simulink model "dfig_dtc_ann"  (R2014a)
settings: Solver=ode23tb  StartTime=0.0  StopTime=10.0  RelTol=1e-3
libraries: neural x106, powerlib x11, powerlib_meascontrol x5, simulink x1
(part 3 of 3)

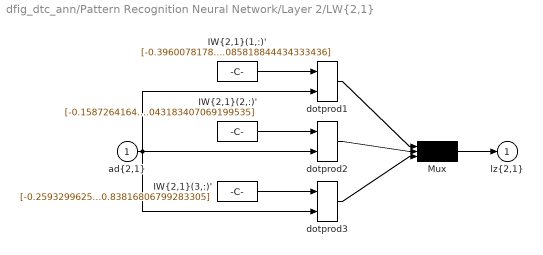
== system dfig_dtc_ann/Pattern Recognition Neural Network/Layer 2/LW{2,1} ==
  "ad{2,1}" : Inport  PortDimensions=100
      mask Display: e = 0.06;c1 = [120 230 180]/255;c2 = ([120 230 180]+0)/(256+128);c3 = ([120 230 180]+128)/(256+128);patch([0 1 1 0],[0 0 1 1],c1);patch([0 1 1 1-e 1-e 0+e],[0 0 1 1-e 0+e 0+e],c2);patch([0 0 1 1-e 0+e 0+e],[0 1 1 1-e 1-e 0+e],c3);plot([0 1 1 0 0],[0 0 1 1 0]);
  "IW{2,1}(1,:)'" : Constant  Value=[-0.39600781788832012;0.80103533096718704;0.41301121989245843;1.1771326908066198;-0.72135382694368677;-0.28776648831982082;0.1961289184675187;1.1440764500026632;-0.23525252157370444;-0.6157189814984334;-0.40248389897597353;-0.4661359120182772;-1.1436532688880334;0.36554497438624434;0.35212901502733357;-1.0882332208589625;0.32805995130326643;-0.37938264281970058;-0.14182705379747199;0.24958969950995402;-0.10265993569030581;0.28425296840325154;-0.32357116420013993;-0.094829576525869916;0.79951067009868138;0.34584911554053616;1.0427282838344432;0.83831785938073644;0.44529056694505259;-0.32121203525474484;0.47873089139593306;0.39423469234562103;-0.13128858500573656;0.92671664955040856;0.045646817038878865;-0.12672354804290886;-0.086421412067187328;0.57657556928792952;-0.062468935112063043;0.26127992146476609;0.34916854352459359;0.39828802839161381;0.76429667962811487;0.22808333560465002;-0.81115136059134063;0.53620443728919553;0.38872445822292429;-0.014891697234410965;0.089173483711878096;0.47345534641936177;-0.71425698724277542;-0.41530443422428559;-0.16469285817743728;-0.37393482186322324;0.18530095941638727;0.64898422181938475;0.09192495445191208;-1.2135091283197963;0.022857999255296524;-0.061188709760653402;0.3432789805346092;0.48379081701553334;-0.11894930315772172;0.017970627109767028;-0.36966997740729218;-0.17616356039153838;0.68742042155939309;0.21297253162193769;0.26859586653067541;-0.37911756178809991;-0.31892610288538376;0.54184108935259523;0.0075175193083964007;-0.29962602080773765;0.56464120152362596;-0.086909709470131366;0.69356886662087025;0.83865301224458633;-0.50614592854819307;-0.1669266161112779;0.61967502129516694;-0.70389310289164331;-0.97647889962465872;0.58839307925056816;-1.2405837996232545;0.30913121120624376;0.44417213686044177;0.85448116388694384;-0.72952901034177886;0.53358762615259592;0.7277496647025159;-0.47770579297136512;0.065512285355189409;-0.024696170024412128;0.33184400224384625;0.77506264674556313;0.14747927143471062;-0.064782569224002454;1.1987950072029985;0.085818844434333436]
      mask Display: e = 0.06;c1 = [120 150 230]/255;c2 = ([120 150 230]+0)/383;c3 = ([120 150 230]+128)/383;patch([0 1 1 0],[0 0 1 1],c1);patch([0 1 1 1-e 1-e 0+e],[0 0 1 1-e 0+e 0+e],c2);patch([0 0 1 1-e 0+e 0+e],[0 1 1 1-e 1-e 0+e],c3);plot([0 1 1 0 0],[0 0 1 1 0]);disp('weights');
  "IW{2,1}(2,:)'" : Constant  Value=[-0.15872641642325955;0.25485844916090572;-0.13632880124207802;-1.0522862221388374;0.012548262724917304;0.050580761236192887;-0.80496802803384571;0.19867650282491883;-0.91745965435057808;-0.84257241706486619;0.065899167127548175;0.54758998719824958;-0.12769643438691047;-0.20898168594609567;-0.64094433173500898;-0.65626789120602724;0.9378120797035765;0.93741066325888078;-0.1115824055347789;0.36549095652773905;0.11096813586489501;0.42307687617734807;-0.36669342329534288;0.82844283524153506;-0.8696511847899131;-0.44266645748114508;-0.21416027683746078;0.11931881155251664;0.82053660406186268;-0.030940761976304361;-0.43271567557985519;1.3438050326709607;0.24153096743304692;0.47835126648124704;-0.72516632400891712;1.0406552999708416;0.53219988971029786;1.6428530389630933;-0.34613733337427577;1.3382882669797933;-0.050102330938810717;0.36085160506818409;0.33183575113754571;-0.21614196040392783;-0.55735322710081481;-0.58225353209158204;0.36550444844041868;0.92056698514446278;-0.26814264333390131;0.64990851258155902;0.6422471733856121;-0.42842320458710942;-0.3550641155339887;0.22066080403826688;-0.48815244166069616;0.72941025675976423;0.51283736806009617;-0.3534937499750086;-1.3312389260991802;-0.39518675849242418;0.78872014932885415;0.35575719119600263;-0.042002321801973025;-1.114402874237632;-0.63378154148624721;-0.23841783841595648;0.56659938013089528;0.20205621739426555;0.19221934898095491;0.11557327779329152;0.75738433485393852;0.82456230330850788;-0.21497552250640226;0.43042182568864623;0.67330144504280764;-0.10709263657939555;0.35267493092517049;0.62842610467547266;-0.33229774822208258;-0.69561342086413736;-0.98378004697372901;-0.17510423116292634;-0.010675115122412697;-0.36995663381985;-0.23043337938054204;-0.13343865366168817;0.39523416686265067;-0.83041390827011785;0.13579111643546179;0.79961703337559364;-0.11902985188294168;-0.099737720935565211;-0.82220442849952646;-0.59133131984649467;-0.013397692495460717;-0.30409995119193683;-0.050800794187225912;-0.58357949953185295;-0.53366952839260839;0.043183407069199535]
      mask Display: e = 0.06;c1 = [120 150 230]/255;c2 = ([120 150 230]+0)/383;c3 = ([120 150 230]+128)/383;patch([0 1 1 0],[0 0 1 1],c1);patch([0 1 1 1-e 1-e 0+e],[0 0 1 1-e 0+e 0+e],c2);patch([0 0 1 1-e 0+e 0+e],[0 1 1 1-e 1-e 0+e],c3);plot([0 1 1 0 0],[0 0 1 1 0]);disp('weights');
  "IW{2,1}(3,:)'" : Constant  Value=[-0.25932996251483764;-0.45562444180686124;0.082585767141114902;0.83272636912942721;0.59433907990150692;0.55001151242535062;-0.56259714883901957;-0.62797492129839039;-0.25938685852771254;-0.058217758000340167;0.044223075395425242;-0.23477610476758989;0.52283195141505323;0.89505974868488569;-0.20701295215162463;0.66816935702873281;0.098098587269625781;0.029573975414518085;0.88218211179692074;0.36073579489144675;-0.40744885981040091;0.092101970169830544;-0.46564910869122011;0.12812380140714019;-1.2827155630720604;0.69695621757152382;0.30812061678832425;0.79767265701525303;0.17672573541318648;-0.54955370831702322;0.033619925789093848;0.49346621662848372;0.56630037710386594;-0.78758323442448408;-0.055222376284757846;0.90928269805545514;-0.12908860635657129;0.42838783825163473;-0.41076812833442228;0.56237657135593522;-0.68700671917372402;-0.64758082415616292;0.99331324379955122;0.23297084258953685;-0.020654675763786677;0.83855505303753397;-0.3252122104798541;0.37193247898627541;-0.10662297511608393;0.51474873965120072;-0.66419405396046727;0.58280501519241523;-0.6526494783117136;0.1216061925420038;-0.078507863021873334;0.28319403079758726;-0.87218346967029692;-0.81577283653680288;-0.41636369589804462;-0.98003924590756508;0.7973673695014436;0.40291242287379286;-0.2867637365923269;0.99759735322669163;0.65834762569595617;1.0678820008485042;-0.23775717257239001;0.084590844274157445;0.41132861031693563;-0.36074025256143272;0.58957921516273259;-0.84150388421390976;-0.33218145349908124;0.23583393588002838;-0.3825655887183963;0.42631617144173894;-0.32964074775802482;0.40295677014248082;0.018782930942609556;-0.66064472557358389;0.79119426329714626;0.37364326884475485;-0.18924863509760317;-0.56498056843220334;-1.0720533763733813;0.59388182732315176;-0.87601519091150082;0.04206405522411967;-0.9920496692258769;0.73122033113882579;-0.08167381081958161;-0.034139549187767876;0.77158401935233578;0.86919728299791199;0.62762726668100355;0.42415120492076525;0.43647371945047997;0.019170076695867701;-0.89256756698482964;-0.83816806799283305]
      mask Display: e = 0.06;c1 = [120 150 230]/255;c2 = ([120 150 230]+0)/383;c3 = ([120 150 230]+128)/383;patch([0 1 1 0],[0 0 1 1],c1);patch([0 1 1 1-e 1-e 0+e],[0 0 1 1-e 0+e 0+e],c2);patch([0 0 1 1-e 0+e 0+e],[0 1 1 1-e 1-e 0+e],c3);plot([0 1 1 0 0],[0 0 1 1 0]);disp('weights');
  Mux : Mux  Inputs=3
      mask Display: e = 0.06;c1 = [120 150 230]/255;c2 = ([120 150 230]+0)/383;c3 = ([120 150 230]+128)/383;patch([0 1 1 0],[0 0 1 1],c1);patch([0 1 1 1-e 1-e 0+e],[0 0 1 1-e 0+e 0+e],c2);patch([0 0 1 1-e 0+e 0+e],[0 1 1 1-e 1-e 0+e],c3);plot([0 1 1 0 0],[0 0 1 1 0]);disp('Mux');
  dotprod1 : neural/Weight Functions/dotprod
  dotprod2 : neural/Weight Functions/dotprod
  dotprod3 : neural/Weight Functions/dotprod
  "lz{2,1}" : Outport
      mask Display: e = 0.06;c1 = [120 230 180]/255;c2 = ([120 230 180]+0)/(256+128);c3 = ([120 230 180]+128)/(256+128);patch([0 1 1 0],[0 0 1 1],c1);patch([0 1 1 1-e 1-e 0+e],[0 0 1 1-e 0+e 0+e],c2);patch([0 0 1 1-e 0+e 0+e],[0 1 1 1-e 1-e 0+e],c3);plot([0 1 1 0 0],[0 0 1 1 0]);
  wires:
  "IW{2,1}(1,:)'"/1 -> dotprod1/1
  "ad{2,1}"/1 -> dotprod1/2, dotprod2/2, dotprod3/2
  dotprod1/1 -> Mux/1
  "IW{2,1}(2,:)'"/1 -> dotprod2/1
  dotprod2/1 -> Mux/2
  "IW{2,1}(3,:)'"/1 -> dotprod3/1
  dotprod3/1 -> Mux/3
  Mux/1 -> "lz{2,1}"/1

== matlab function dfig_dtc_ann/Two-Level Hystereis Band ==
  data: FluxRef input; Hf output; Flux input; m input; mm output
function [Hf,mm] = Two_Level_Hys(FluxRef,Flux,m)
 
DelF=0.025;% Hysteresis Width for Flux
Hf=0;%Initializing Hysteresis Controller Output For Flux
mm=m;
% Flux Two Level Hysteresis Band %
%------------------------------------------------------------------------%
if(Flux<=(FluxRef-DelF))
    Hf=1;
    mm=Hf;
end
if(mm==1&&(Flux>(FluxRef-DelF))&&(Flux<(FluxRef+DelF)))
    Hf=1;
    mm=Hf;
end
if(Flux>=(FluxRef+DelF))
    Hf=0;
    mm=Hf;
end
if(mm==0&&(Flux>(FluxRef-DelF))&&(Flux<(FluxRef+DelF)))
    Hf=0;
    mm=Hf;
end

== matlab function dfig_dtc_ann/Rotor Flux Torque Estimator (4) ==
  data: Sird input; SirMag output; Sirq input; Irq input; Sisd input; SirAng output; Torque output
function [SirMag,SirAng,Torque] = Rotor_Flux_Torque_Estimator(Sird,Sirq,Irq,Sisd)
 SirMag=((Sird)^(2)+(Sirq)^(2))^(0.5);
 x=atan2(Sirq,Sird);
 if(x>=0)
    SirAng=x*(180/pi);
 else
    SirAng=x*(180/pi)+360;
 end
 Torque=(-3)*(0.0135/0.0136)*(Sisd*Irq);

== matlab function dfig_dtc_ann/Stator Flux Estimator (2) ==
  settings: updateMethod=CONTINUOUS
  data: Sisd input; SiMag output; Sisq input; SiAng output
function [SiMag,SiAng] = StatorFlux_MagAng_Estimator(Sisd,Sisq)
 SiMag=((Sisd)^(2)+(Sisq)^(2))^(0.5);
 x=atan2(Sisq,Sisd);
 if(x>=0)
    SiAng=x;
 else
    SiAng=x+(2*pi);
 end

== matlab function dfig_dtc_ann/Three-Level Hystereis Band ==
  data: TorqueRef input; Ht output; Torque input; m input; mm output
function [Ht,mm] = Three_Level_Hys(TorqueRef,Torque,m)
 
DelT=0.025;% Hysteresis Width for Torque
Ht=0;%Initializing Hysteresis Controller Output For Torque
mm=m;

% Torque Three Level Hysteresis Band %
%------------------------------------------------------------------------%
if(Torque<=(TorqueRef-DelT))
    Ht=1;
    mm=Ht;
end
if((Torque>(TorqueRef-DelT))&&(Torque<TorqueRef)&&mm==1)
    Ht=1;
    mm=Ht;
end
if(Torque>=(TorqueRef+DelT))
    Ht=-1;
    mm=Ht;
end
if((Torque<(TorqueRef+DelT))&&(Torque>TorqueRef)&&mm==-1)
    Ht=-1;
    mm=Ht;
end
if((Torque>(TorqueRef-DelT))&&(Torque<TorqueRef)&&mm==-1)
    Ht=0;
    mm=-1;
end
if((Torque<(TorqueRef+DelT))&&(Torque>TorqueRef)&&mm==1)
    Ht=0;
    mm=1;
end

== matlab function dfig_dtc_ann/Rotor Flux Sector ==
  data: FluxAng input; S output; Wr input; W output
function [S,W]= Rotor_Flux_Sector(FluxAng,Wr)
 
S=0;
W=0;

if(Wr<=(50*pi))
    W=1;
else
    W=0;
end
% DTC Sector Prediction %
%------------------------------------------------------------------------%
if(FluxAng>=330&&FluxAng<30)
    S=1;
end
if(FluxAng>=30&&FluxAng<90)
    S=2;
end
if(FluxAng>=90&&FluxAng<150)
    S=3;
end
if(FluxAng>=150&&FluxAng<210)
    S=4;
end
if(FluxAng>=210&&FluxAng<270)
    S=5;
end
if(FluxAng>=270&&FluxAng<330)
    S=6;
end

== matlab function dfig_dtc_ann/Neural Net Corrector ==
  data: x1 input; x3 input; T1 output; x5 input; T3 output; T5 output
function [T1,T3,T5] = NeuralNet_Corrector(x1,x3,x5)

if(x1>=0.2)
    T1=1;
else
    T1=0;
end
if(x3>=0.2)
    T3=1;
else
    T3=0;
end
if(x5>=0.2)
    T5=1;
else
    T5=0;
end
